simulink model "elavtor_model"  (R2020a)
settings: Solver=VariableStepAuto  StartTime=0.0  StopTime=10.0  RelTol=1e-3
settings Model: Creator=INDRAJIT MARATHE  LastModifiedBy=INDRAJIT MARATHE

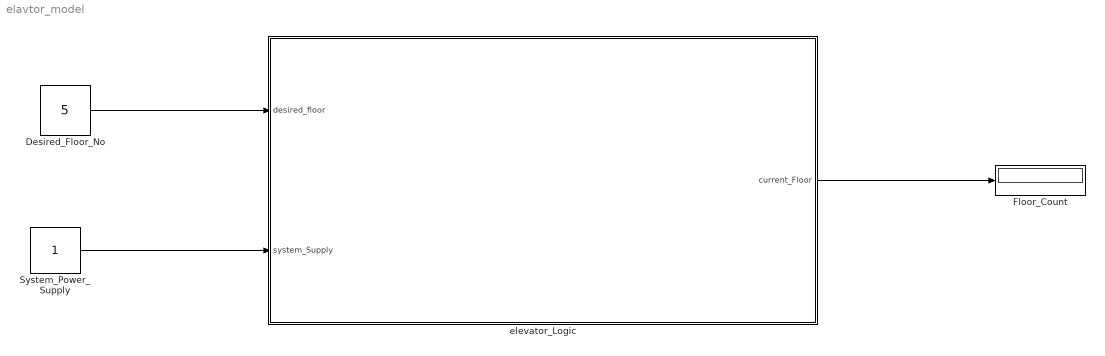
== system elavtor_model ==
  Desired_Floor_No : Constant  Value=5
  Floor_Count : Display
  System_Power_Supply : Constant
  elevator_Logic : Stateflow chart  TreatAsAtomicUnit=on
  wires:
  Desired_Floor_No/1 -> elevator_Logic/1(desired_floor)
  System_Power_Supply/1 -> elevator_Logic/2(system_Supply)
  elevator_Logic/1(current_Floor) -> Floor_Count/1

== stateflow chart elavtor_model/elevator_Logic ==
  state elevator_OnOff_state [parallel]
    settings: executionOrder=1
    state Idle
      current_Floor=0;
    state Active
    (default) -> Idle : {current_Floor=1;}
    Idle -> Active : [system_Supply ==1]
    Active -> Idle : [system_Supply==0]
  state elevator_Run_state [parallel]
    settings: executionOrder=2
    state goUP_floor
      du:
      current_Floor=current_Floor+1;
    state entrance_logic
    state goDOWN_floor
      du:
      current_Floor=current_Floor-1;
    state Wait
    (default) -> entrance_logic
    entrance_logic -> goUP_floor [order 2] : [desired_floor>current_Floor]
    entrance_logic -> goDOWN_floor [order 1] : [desired_floor<current_Floor]
    goUP_floor -> Wait : [current_Floor==desired_floor]
    Wait -> entrance_logic : after(3,sec)
    goDOWN_floor -> Wait : [current_Floor==desired_floor]
  (default) -> elevator_OnOff_state
  data: desired_floor input; system_Supply input; current_Floor output
